simulink model "offcentercriterion"  (R2024a)
settings: Solver=VariableStepAuto  StartTime=0.0  StopTime=50  RelTol=1e-3
values from neighbouring files (symbols this model uses):
  b = b_values(i)    [firstharmonicbodeplots.m]    (also in stabilitycriterions.m = -0.5; untitled.m)
settings Model: Creator=Hp  LastModifiedBy=Hp

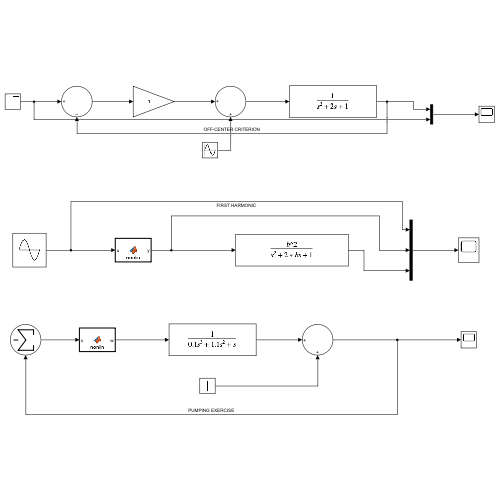
[thumbnail: Simulink's stored preview of the top-level diagram]
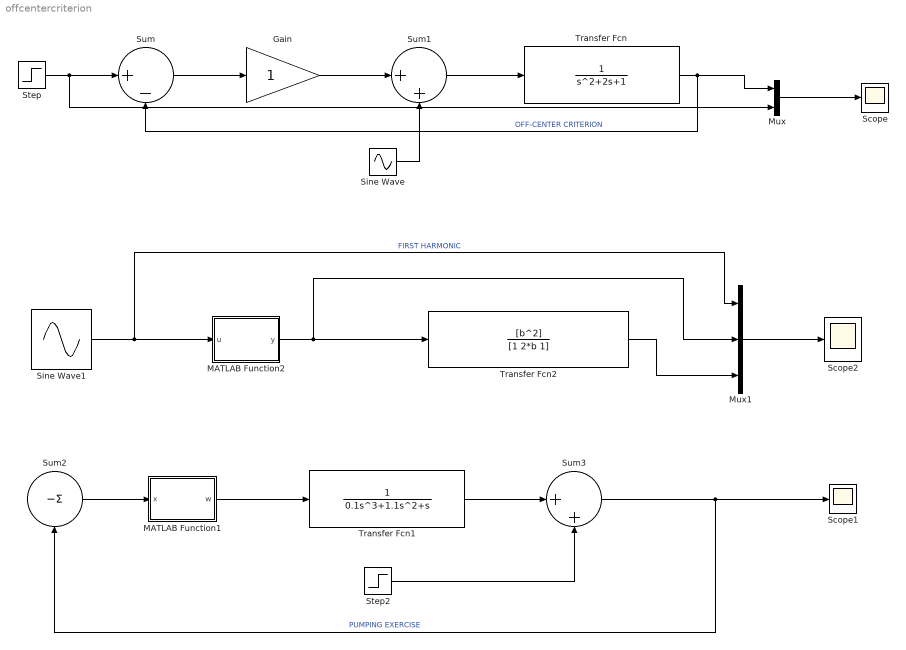
== system offcentercriterion ==
  Gain : Gain
  MATLAB Function1 : MATLAB Function  TreatAsAtomicUnit=on
  MATLAB Function2 : MATLAB Function  TreatAsAtomicUnit=on
  Mux : Mux  Inputs=2
  Mux1 : Mux  Inputs=3
  Scope : Scope
  Scope1 : Scope
  Scope2 : Scope
  Sine Wave : Sin  SampleTime=0
  Sine Wave1 : Sin  Frequency=5  SampleTime=0
  Step : Step  Time=0  SampleTime=0
  Step2 : Step  Time=0  After=12  SampleTime=0
  Sum : Sum  Inputs=|+-
  Sum1 : Sum  Inputs=|++
  Sum2 : Sum  Inputs=|-
  Sum3 : Sum  Inputs=|++
  Transfer Fcn : TransferFcn
  Transfer Fcn1 : TransferFcn  Denominator=[0.1 1.1 1 0]
  Transfer Fcn2 : TransferFcn  Numerator=[b^2]  Denominator=[1 2*b 1]
  wires:
  Step/1 -> Mux/2, Sum/1
  Sum/1 -> Gain/1
  Gain/1 -> Sum1/1
  Sum1/1 -> Transfer Fcn/1
  Sine Wave/1 -> Sum1/2
  Transfer Fcn/1 -> Mux/1, Sum/2  "OFF-CENTER CRITERION"
  Mux/1 -> Scope/1
  MATLAB Function1/1(w) -> Transfer Fcn1/1
  Sum2/1 -> MATLAB Function1/1(x)
  Transfer Fcn1/1 -> Sum3/1
  Sum3/1 -> Scope1/1, Sum2/1  "PUMPING EXERCISE"
  Step2/1 -> Sum3/2
  Sine Wave1/1 -> MATLAB Function2/1(u), Mux1/1  "FIRST HARMONIC"
  MATLAB Function2/1(y) -> Mux1/2, Transfer Fcn2/1
  Transfer Fcn2/1 -> Mux1/3
  Mux1/1 -> Scope2/1

== matlab function offcentercriterion/MATLAB Function2 ==
  data: u input; y output
function y = nonlin(u)
k=2;
a=1;
    if u > a
        y = k*a;      % saturate at +k*a
    elseif u < -a
        y = -k*a;     % saturate at -k*a
    else
        y = k*u;      % linear region
    end
end

== matlab function offcentercriterion/MATLAB Function1 ==
  data: x input; w output
function w = nonlin(x)
M = 10;
xm = 1;
k = M/xm;

if abs(x) <= xm
    w = k*x;
else
    w = M*sign(x);
end
